simulink library "csu_lic_landing_inter_coast_lib"  (R2014b)
settings: Solver=ode45  StartTime=0.0  StopTime=10.0  RelTol=1e-3
values from neighbouring files (symbols this model uses):
  lic_coast_complete_altitude = 8000    [csu_lic_landing_inter_coast_init.m]
libraries: util_info_lib x1, simulink x1
settings Model: Creator=escrane  LastModifiedBy=mstewart

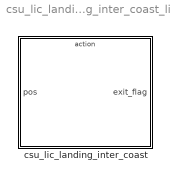
== system csu_lic_landing_inter_coast_lib ==
  csu_lic_landing_inter_coast : Subsystem  TreatAsAtomicUnit=on

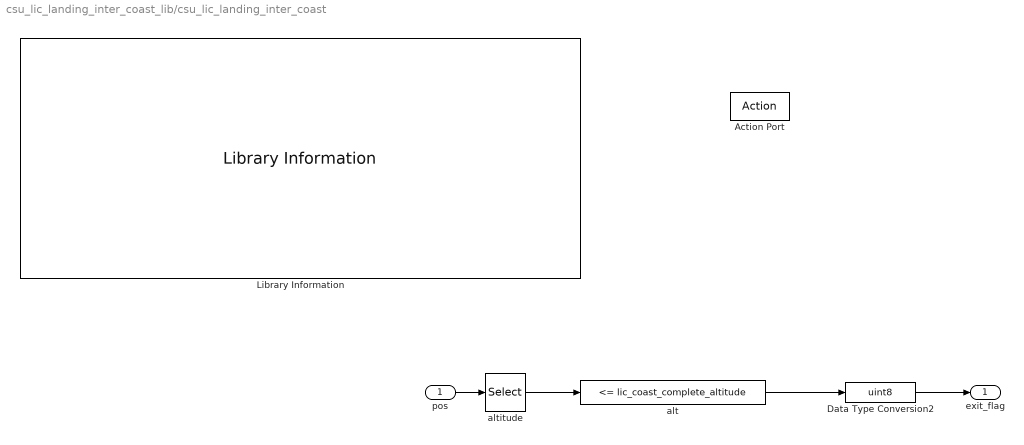
== system csu_lic_landing_inter_coast_lib/csu_lic_landing_inter_coast ==
  pos : Inport
  Action Port : ActionPort
  Data Type Conversion2 : DataTypeConversion  OutDataTypeStr=uint8
  Library Information : util_info_lib/Library Information  owner='NONE'
  alt : simulink/Logic and Bit Operations/Compare To Constant  relop=<=  const=lic_coast_complete_altitude  OutDataTypeStr=boolean
  altitude : Selector  InputPortWidth=3  Indices=[3]
  exit_flag : Outport  InitialOutput=0
  wires:
  Data Type Conversion2/1 -> exit_flag/1
  alt/1 -> Data Type Conversion2/1
  altitude/1 -> alt/1
  pos/1 -> altitude/1
